simulink model "parte4_eje3_Thidraulica_mdl"  (R2017b)
settings: Solver=VariableStepAuto  StartTime=0.0  StopTime=50  RelTol=1e-3
values from neighbouring files (symbols this model uses):
  At = 1/(gFL-gNL)    (= 1.25)    [parte4_ej1_ThidraulicaNLdata.m]    (also in parte4_eje2_Thidraulica_const.m)
  CI = 10    [parte4_eje2_Thidraulica_const.m]
  Ho = 1    [parte4_ej1_ThidraulicaNLdata.m]    (also in parte4_eje2_Thidraulica_const.m)
  PR = 1    [parte4_eje2_Thidraulica_const.m]
  R = 0.05    [parte4_eje2_Thidraulica_const.m]
  r = 0.1    [parte4_eje2_Thidraulica_const.m]
  Tf = 0.05    [parte4_eje2_Thidraulica_const.m]
  Tg = 0.5    [parte4_eje2_Thidraulica_const.m]
  Tr = 5    [parte4_eje2_Thidraulica_const.m]
  TW = 1    [parte4_ej1_ThidraulicaNLdata.m]    (also in parte4_eje2_Thidraulica_const.m)
  UNL = 0.068    [parte4_ej1_ThidraulicaNLdata.m]    (also in parte4_eje2_Thidraulica_const.m = 0.08)
  w = 1    [parte4_ej1_ThidraulicaNLdata.m]    (also in parte4_eje2_Thidraulica_const.m)
settings Model: Creator=cjuar  LastModifiedBy=Admon

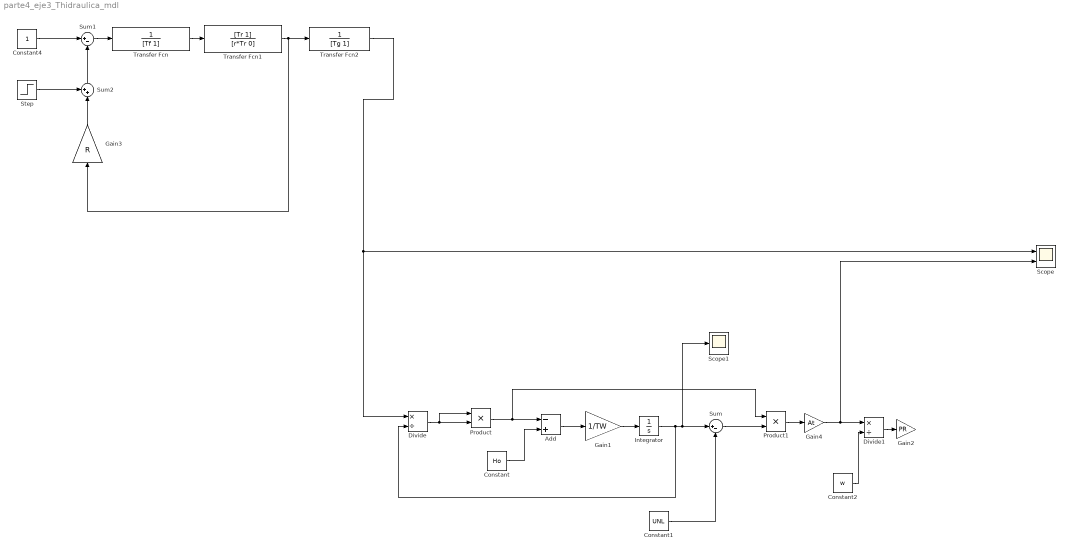
== system parte4_eje3_Thidraulica_mdl ==
  Add : Sum  Inputs=-+
  Constant : Constant  Value=Ho
  Constant1 : Constant  Value=UNL
  Constant2 : Constant  Value=w
  Constant4 : Constant
  Divide : Product  Inputs=*/
  Divide1 : Product  Inputs=*/
  Gain1 : Gain  Gain=1/TW
  Gain2 : Gain  Gain=PR
  Gain3 : Gain  Gain=R
  Gain4 : Gain  Gain=At
  Integrator : Integrator  InitialCondition=CI  UpperSaturationLimit=10
  Product : Product
  Product1 : Product
  Scope : Scope  NumInputPorts=2
  Scope1 : Scope
  Step : Step  Before=1  After=1.1  SampleTime=0
  Sum : Sum  Inputs=|+-
  Sum1 : Sum  Inputs=|+-
  Sum2 : Sum  Inputs=++|
  Transfer Fcn : TransferFcn  Denominator=[Tf 1]
  Transfer Fcn1 : TransferFcn  Numerator=[Tr 1]  Denominator=[r*Tr 0]
  Transfer Fcn2 : TransferFcn  Denominator=[Tg 1]
  wires:
  Transfer Fcn2/1 -> Divide/1, Scope/1
  Divide/1 -> Product/1, Product/2
  Product/1 -> Product1/1, Add/1
  Constant/1 -> Add/2
  Add/1 -> Gain1/1
  Gain1/1 -> Integrator/1
  Constant1/1 -> Sum/2
  Sum/1 -> Product1/2
  Constant2/1 -> Divide1/2
  Divide1/1 -> Gain2/1
  Product1/1 -> Gain4/1
  Transfer Fcn/1 -> Transfer Fcn1/1
  Transfer Fcn1/1 -> Transfer Fcn2/1, Gain3/1
  Sum1/1 -> Transfer Fcn/1
  Sum2/1 -> Sum1/2
  Gain3/1 -> Sum2/2
  Constant4/1 -> Sum1/1
  Step/1 -> Sum2/1
  Integrator/1 -> Scope1/1, Sum/1, Divide/2
  Gain4/1 -> Scope/2, Divide1/1
